simulink model "demo_20210521"  (Simulink 7.9)
settings: Solver=FixedStepDiscrete  StartTime=0.0  StopTime=0  RelTol=1e-3
undefined symbols (not defined in the file or in its folder): jet
libraries: visionsinks x2, visionconversions x1, visionsources x1
settings Model: Creator=thinkpad  LastModifiedBy=thinkpad

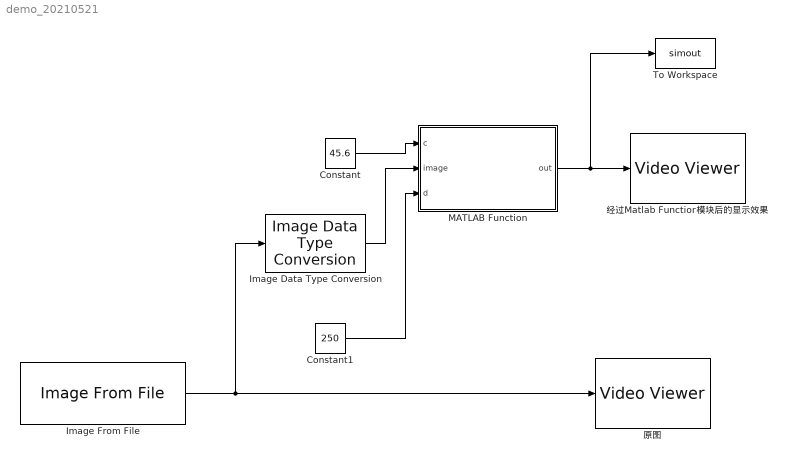
== system demo_20210521 ==
  Constant : Constant  Value=45.6
  Constant1 : Constant  Value=250
  Image Data Type Conversion : visionconversions/Image Data Type Conversion  outDT=single  isSigned=on  wordLen=16  numFracBits=0
  Image From File : visionsources/Image From File  Tag=vipblks_nd  FileName=cameraman.tif  imagePorts=One multidimensional signal  Ts=inf  ImageDataType=Inherit from input image  Signed=on  WordLength=16  sdImageDataType=uint(8)  FractionLengthMode=User-defined  FractionLength=15  OutPortLabels=R|G|B
  MATLAB Function : MATLAB Function  TreatAsAtomicUnit=on
  To Workspace : ToWorkspace  VariableName=simout  SampleTime=-1  SaveFormat=Timeseries
  原图 : visionsinks/Video Viewer  inputType=Obsolete7b  imagePorts=One multidimensional signal  useColorMap=off  colormapValue=jet(256)  specRange=off  minInputVal=0  maxInputVal=255  FigPos=[85 544 410 293]  AxisZoom=on  trueSizedOnce=off  OpenAtMdlStart=on
  经过Matlab Function模块后的显示效果 : visionsinks/Video Viewer  inputType=Obsolete7b  imagePorts=One multidimensional signal  useColorMap=off  colormapValue=jet(256)  specRange=off  minInputVal=0  maxInputVal=255  FigPos=[594 565 410 306]  AxisZoom=on  trueSizedOnce=off  OpenAtMdlStart=on
  wires:
  Constant/1 -> MATLAB Function/1(c)
  MATLAB Function/1(out) -> 经过Matlab Function模块后的显示效果/1, To Workspace/1
  Image From File/1 -> 原图/1, Image Data Type Conversion/1
  Image Data Type Conversion/1 -> MATLAB Function/2(image)
  Constant1/1 -> MATLAB Function/3(d)

== matlab function MATLAB Function ==
  data: c input double; out output double; image input double; d input double
function out = fcn(c, image, d)
out = log(abs(fftshift(fft2(c + d + double(image)))));
% out = (image > c);
